simulink subsystem "V4_Modell_EM"  (R2022b)
settings: Solver=VariableStepAuto  StartTime=0.0  StopTime=10.0  RelTol=1e-3
values from neighbouring files (symbols this model uses):
  k_M = C_Phi    (= 42.43)    [V4_Parameter_Parameter_komplett_te.m]    (also in V4_Parameter_Wagen_Te.m = -0.04243; V4_Parameter_komplett.m = -0.04243)
  KL_R_VH = [10 20 30 40; 0.57 0.2905 0.255 0.207]    [V4_Parameter_EM.m]    (also in V4_Parameter_Parameter_komplett_te.m; V4_Parameter_komplett.m)
settings Model: Creator=JSCHB  LastModifiedBy=Patrick

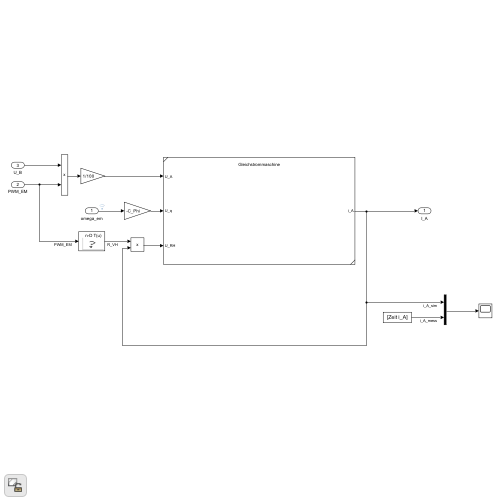
[thumbnail: Simulink's stored preview of the top-level diagram]
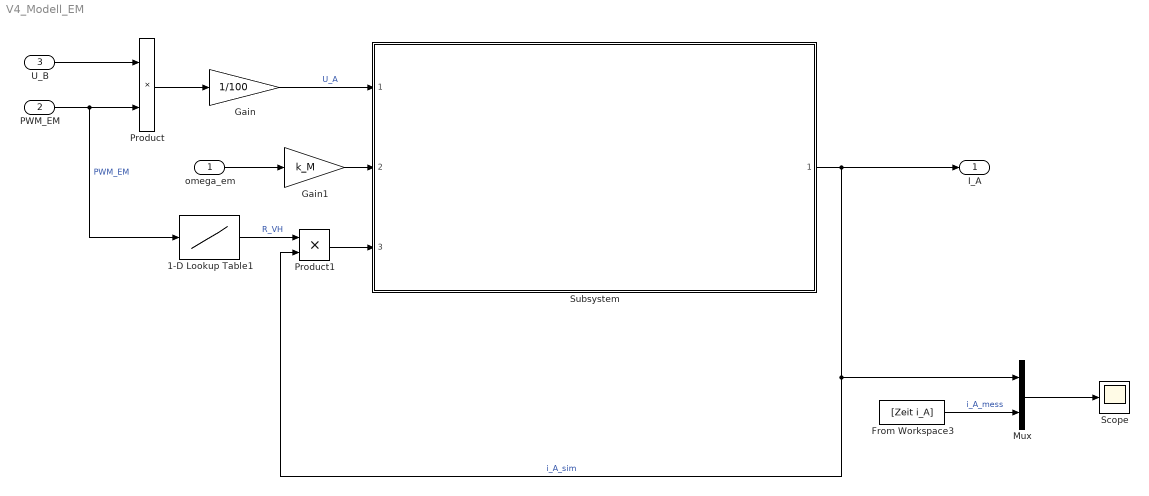
== system V4_Modell_EM ==
  omega_em : Inport
  PWM_EM : Inport  Port=2
  U_B : Inport  Port=3
  1-D Lookup Table1 : Lookup_n-D  NumberOfTableDimensions=1  BreakpointsForDimension1=KL_R_VH(1,:)  Table=KL_R_VH(2,:)  InternalRulePriority=Speed  RndMeth=Simplest
  From Workspace3 : FromWorkspace  VariableName=[Zeit i_A]
  Gain : Gain  Gain=1/100
  Gain1 : Gain  Gain=k_M
  Mux : Mux  Inputs=2
  Product : Product
  Product1 : Product
  Scope : Scope
  Subsystem : Subsystem  ReferencedSubsystem=Gleichstrommaschine
  I_A : Outport
  wires:
  From Workspace3/1 -> Mux/2  "i_A_mess"
  Product1/1 -> Subsystem/3
  1-D Lookup Table1/1 -> Product1/1  "R_VH"
  Subsystem/1 -> I_A/1, Product1/2, Mux/1  "i_A_sim"
  Gain/1 -> Subsystem/1  "U_A"
  PWM_EM/1 -> Product/2, 1-D Lookup Table1/1  "PWM_EM"
  Product/1 -> Gain/1
  Gain1/1 -> Subsystem/2
  Mux/1 -> Scope/1
  U_B/1 -> Product/1
  omega_em/1 -> Gain1/1
